simulink model "EarthPointingGuidance_JackGuidance"  (R2019b)
settings: Solver=FixedStepAuto  StartTime=0.0  StopTime=31622400  FixedStep=60  RelTol=1e-3
InitFcn:
  | RWPJ06_init_param
  | load('B5G_inclin_29.mat')
settings Model: SimulationMode=accelerator  Creator=b0301  LastModifiedBy=b0301
settings DataIOCC: ReturnWorkspaceOutputs=off

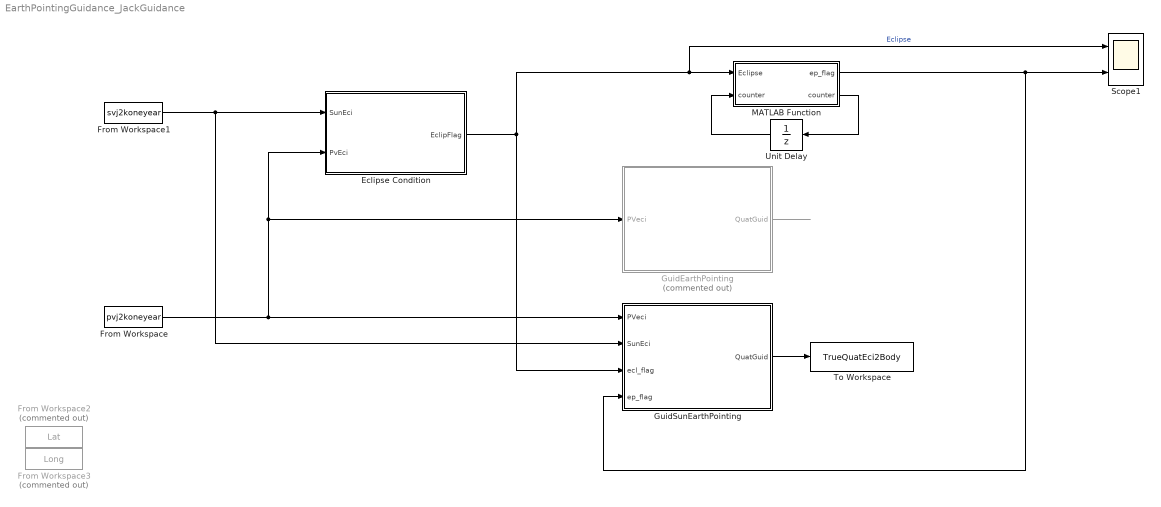
== system EarthPointingGuidance_JackGuidance ==
  Eclipse Condition : MATLAB Function  TreatAsAtomicUnit=on
  From Workspace : FromWorkspace  VariableName=pvj2koneyear  SampleTime=0
  From Workspace1 : FromWorkspace  VariableName=svj2koneyear  SampleTime=0
  From Workspace2 : FromWorkspace  Commented=on  VariableName=Lat  SampleTime=0
  From Workspace3 : FromWorkspace  Commented=on  VariableName=Long  SampleTime=0
  GuidEarthPointing : MATLAB Function  Commented=on  TreatAsAtomicUnit=on
  GuidSunEarthPointing : MATLAB Function  TreatAsAtomicUnit=on
  MATLAB Function : MATLAB Function  TreatAsAtomicUnit=on
  Scope1 : Scope  NumInputPorts=2
  To Workspace : ToWorkspace  VariableName=TrueQuatEci2Body  SaveFormat=Timeseries  SampleTime=-1
  Unit Delay : UnitDelay  SampleTime=-1  HasFrameUpgradeWarning=on
  wires:
  From Workspace/1 -> GuidEarthPointing/1(PVeci), Eclipse Condition/2(PvEci), GuidSunEarthPointing/1(PVeci)
  GuidEarthPointing/1(QuatGuid) -> ?
  From Workspace1/1 -> GuidSunEarthPointing/2(SunEci), Eclipse Condition/1(SunEci)
  Eclipse Condition/1(EclipFlag) -> GuidSunEarthPointing/3(ecl_flag), Scope1/1, MATLAB Function/1(Eclipse)  "Eclipse"
  GuidSunEarthPointing/1(QuatGuid) -> To Workspace/1
  MATLAB Function/1(ep_flag) -> GuidSunEarthPointing/4(ep_flag), Scope1/2
  MATLAB Function/2(counter) -> Unit Delay/1
  Unit Delay/1 -> MATLAB Function/2("counter ")

== matlab function EarthPointingGuidance_JackGuidance/GuidSunEarthPointing ==
  data: PVeci input; SunEci input; QuatGuid output; ecl_flag input; ep_flag input
function QuatGuid = EarthSunPointingGuid(PVeci, SunEci, ecl_flag, ep_flag) %, lat, long
sun_flag = ~ecl_flag;
Qi2l     = PVi2Qi2l(PVeci);

if sun_flag == 0 %% eclipse, earth pointing
    QuatGuid  = Qi2l;
else
    
%     SunBody   = SS_TM(1:3);
%     SunEci    = FrameA2B(SunBody,  QInv(Qi2b)); % body to eci
    OrbNrmEci = FrameA2B([0 -1 0]', QInv(Qi2l)); % lvlh to eci
    SunOrbitRelation = dot(OrbNrmEci,SunEci);
    
    if 1 %(SunOrbitRelation > 0) %% Sun Vector and Orbit Normal at same side
        Ur = cross(cross(OrbNrmEci,SunEci),SunEci);
        Uz = -SunEci;
        if 0 % decending
            Ux = Ur;
%         Ux = cross(OrbNrmEci,SunEci);
%             Uz = -SunEci;
            Uy = cross(Uz,Ux);
        else % ascending
            Uy = Ur;
%         Ux = cross(OrbNrmEci,SunEci);
%             Uz = -SunEci;
            Ux = cross(Uy,Uz);
        end
    else %% Sun Vector and Orbit Normal at different side
        Ux = -cross(cross(OrbNrmEci,SunEci),SunEci);
%         Ux = cross(OrbNrmEci,SunEci);
        Uz = -SunEci;
        Uy = cross(Uz,Ux);
    end
    
    QuatGuid  = M2Q([Ux Uy Uz]);
    
    gap = Qi2l;
    sup = QuatGuid;
    
    signflip=[0 0 0 1;0 0 -1 0; 0 1 0 0;-1 0 0 0];
    a1 = gap'*(signflip*sup);
    b1 = gap'*sup;
    theta   = atan2(-a1,b1);
    
    sup_com = [cos(theta) 0 0 sin(theta)]';
    new_sup = QMul(sup, sup_com);
    
    QuatGuid = new_sup;
    
%     getAxErr(gap, sup);
%     fprintf('\n--new sup--');
%     getAxErr(gap, new_sup);
    
    
%     OmegaGuid = zeros(3,1);
end


end

% 
% function [eigAng, AxAngs] = getAxErr(Qa, Qb)
% deltaQ = QMul(QInv(Qa),Qb);
% if deltaQ(1)<0
%         deltaQ = deltaQ *-1;
% end
%     AxAngs = 2.0*deltaQ(2:4)*180/pi;
%     eigAng = 2*atan2d(norm(deltaQ(2:4)),deltaQ(1));
%     fprintf('\neigAng \t\t= %.2f deg\nAxisError \t= [%.2f %.2f %.2f] deg\n',eigAng,AxAngs);
% end

== matlab function EarthPointingGuidance_JackGuidance/MATLAB Function ==
  data: Eclipse input; ep_flag output; counter input; counter output
function [ep_flag,counter] = fcn(Eclipse,counter)
ep_flag = 0;
dt = 60;

if ~Eclipse
    counter = counter+dt;
    if counter >1246 && counter < 1246*2
        ep_flag = 1;
    else
        ep_flag = 0;
    end
else
    counter = 0;
end

== matlab function EarthPointingGuidance_JackGuidance/GuidEarthPointing ==
  data: PVeci input; QuatGuid output
function QuatGuid = EarthPointingGuidance(PVeci)
QuatGuid  = PVi2Qi2l(PVeci);
end

== matlab function EarthPointingGuidance_JackGuidance/Eclipse Condition ==
  data: SunEci input; EclipFlag output; PvEci input
function EclipFlag  = Eclipse(SunEci, PvEci)
Dp = -PvEci(1:3)*1e-3;  % earth vector in Km
Rp = 6378.137;          % earth radius in km
Rs = 6.9599e5;          % solar photosphere radius in km
S  = 1.49597870e8;      % astronomical unit in km
C  = 1.385e6;           % size of earth shadow cone
Ds = (S.*SunEci + Dp);  % vector from S/C to the Sun
 
DsNorm = norm(Ds);
DpNorm = norm(Dp);
rho_s  = asind(Rs/DsNorm);
rho_p  = asind(Rp/DpNorm);
theta  = acosd(dot(Ds, Dp) / (DsNorm * DpNorm));
if ( theta < (rho_p - rho_s) && DsNorm > S && (S + C) > DsNorm)
    EclipFlag = 1;
else
    EclipFlag = 0;
end
